simulink model "Counters"  (R2020a)
settings: Solver=VariableStepAuto  StartTime=0.0  StopTime=10.0  RelTol=1e-3
libraries: simulink x1
settings Model: Creator=ashok  LastModifiedBy=ashok

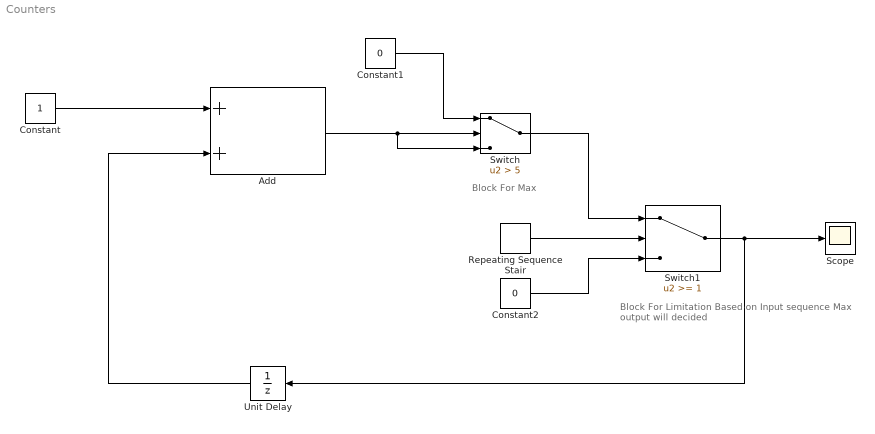
== system Counters ==
  note: Block For Limitation
      | Based on Input sequence Max output will decided
  note: Block For Max
  Add : Sum
  Constant : Constant
  Constant1 : Constant  Value=0
  Constant2 : Constant  Value=0
  Repeating Sequence Stair : simulink/Sources/Repeating Sequence Stair  OutValues=[1 1 1 0 0 0 1 1 1 1 1 0 0 0 0 ].'  tsamp=-1  OutMin=[]  OutMax=[]  OutDataTypeStr=double  OutputDataTypeScalingMode=double  OutDataType=fixdt(0,8)  ConRadixGroup=Best Precision: Vector-wise  OutScaling=2^-12
  Scope : Scope
  Switch : Switch  Criteria=u2 > Threshold  Threshold=5
  Switch1 : Switch  Threshold=1
  Unit Delay : UnitDelay  SampleTime=-1  HasFrameUpgradeWarning=on
  wires:
  Constant/1 -> Add/1
  Unit Delay/1 -> Add/2
  Add/1 -> Switch/3, Switch/2
  Constant1/1 -> Switch/1
  Switch/1 -> Switch1/1
  Repeating Sequence Stair/1 -> Switch1/2
  Constant2/1 -> Switch1/3
  Switch1/1 -> Scope/1, Unit Delay/1
